simulink library "Lib_Turbo_Inlet_TMATS"  (R2012b)
settings: Solver=ode45  StartTime=0.0  StopTime=10.0  RelTol=1e-3
Description:
  | Thomas Modules
settings Model: Creator=jwchapm2  LastModifiedBy=jwchapm2

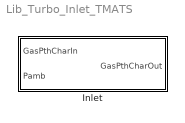
== system Lib_Turbo_Inlet_TMATS ==
  Inlet : Subsystem  mask(T-MATS: Inlet Library Block){eRambase_M=1, X_eRamVec_M=[0 3], T_eRamtbl_M=[1 1]}
      mask prompts: eRambase_M "eRambase_M - Base delta pressure [frac]"; X_eRamVec_M "X_eRamVec_M - Pt/Pamb Vector [nx1]"; T_eRamtbl_M "T_eRamtbl_M - delta pressure based on Pt/Pamb [frac][nx1)"
      mask help: This block simulates the performance of an inlet using basic fluid dynamic equations and properties.
      mask Help: web(which('Turbo_TMATS_Inlet.html'),'-helpbrowser')

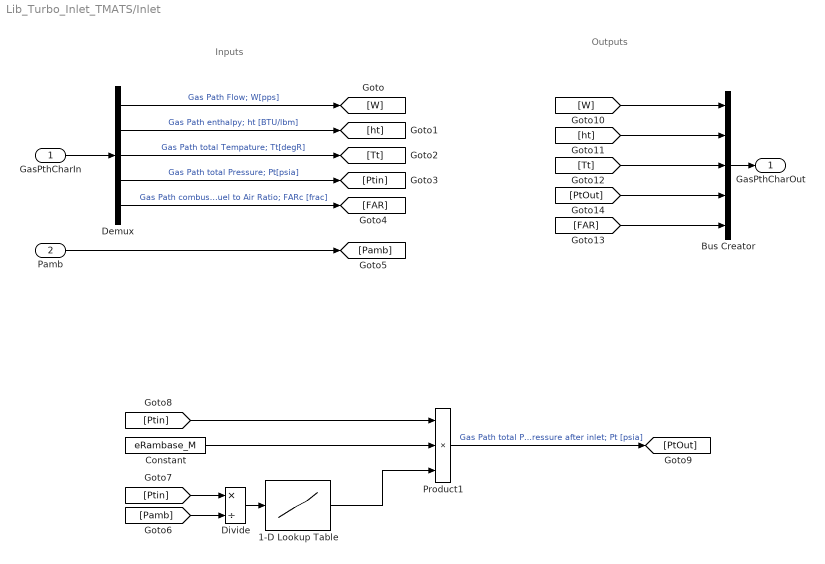
== system Lib_Turbo_Inlet_TMATS/Inlet ==
  note: Inputs
  note: Outputs
  GasPthCharIn : Inport
  Pamb : Inport  Port=2
  1-D Lookup Table : Lookup_n-D  NumberOfTableDimensions=1  BreakpointsForDimension1=X_eRamVec_M  Table=T_eRamtbl_M  ExtrapMethod=Clip  DiagnosticForOutOfRangeInput=Warning  UseLastTableValue=on  RndMeth=Simplest  InputSameDT=on
  Bus Creator : BusCreator  Inputs=5
  Constant : Constant  Value=eRambase_M
  Demux : Demux  Outputs=5
  Divide : Product  Inputs=*/
  Product1 : Product  Inputs=3  RndMeth=Zero
  GasPthCharOut : Outport
  wires:
  Demux/1 -> [W]  "Gas Path Flow; W[pps]"
  Demux/5 -> [FAR]  "Gas Path combusted Fuel to Air Ratio; FARc [frac]"
  Demux/3 -> [Tt]  "Gas Path total Tempature; Tt[degR]"
  GasPthCharIn/1 -> Demux/1
  Bus Creator/1 -> GasPthCharOut/1
  Product1/1 -> [PtOut]  "Gas Path total Pressure after inlet; Pt [psia]"
  Demux/4 -> [Ptin]  "Gas Path total Pressure; Pt[psia]"
  Demux/2 -> [ht]  "Gas Path enthalpy; ht [BTU/lbm]"
  Pamb/1 -> [Pamb]
  [Ptin] -> Divide/1
  [Pamb] -> Divide/2
  Divide/1 -> 1-D Lookup Table/1
  [Ptin] -> Product1/1
  Constant/1 -> Product1/2
  1-D Lookup Table/1 -> Product1/3
  [FAR] -> Bus Creator/5
  [Tt] -> Bus Creator/3
  [ht] -> Bus Creator/2
  [W] -> Bus Creator/1
  [PtOut] -> Bus Creator/4
